simulink model "derivativemanuevermissile"  (Simulink 10.0)
settings: Solver=ode23t  StartTime=0.0  StopTime=20  RelTol=1e-3  EnableMultiTasking=on
StopFcn:
  | startplot
settings Model: Creator=Admin  LastModifiedBy=asuresh4
settings DataIOCC: LimitDataPoints=on  SignalLoggingSaveFormat=ModelDataLogs
settings OptimizationCC: ExpressionDepthLimit=2147483647
settings DebuggingCC: FcnCallInpInsideContextMsg=warning  StateNameClashWarn=warning
settings ConfigComp: CovExternalEMLEnable=off

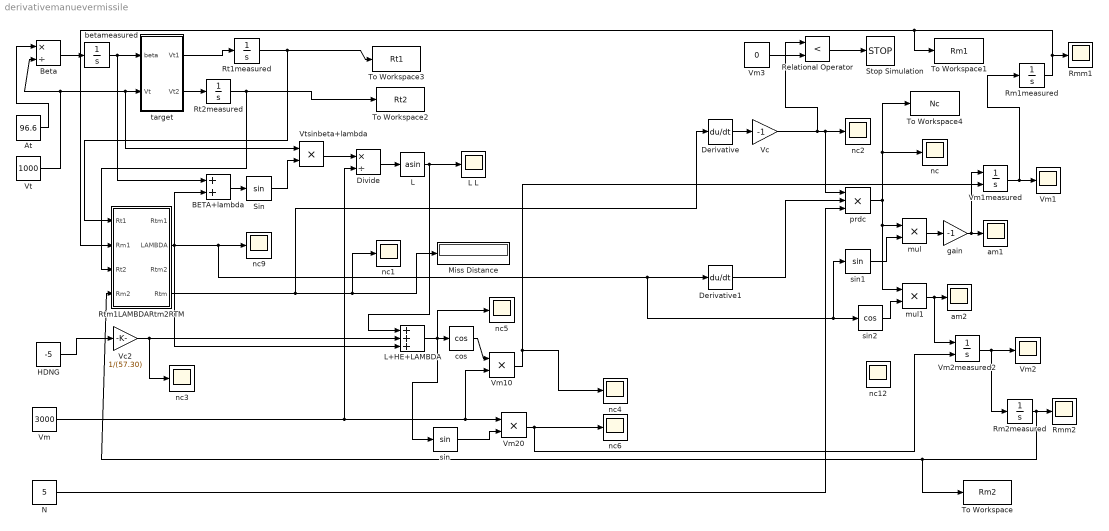
== system derivativemanuevermissile ==
  At : Constant  Value=96.6
  BETA+lambda : Sum
  Beta : Product  Inputs=*/
  Derivative : Derivative
  Derivative1 : Derivative
  Divide : Product  Inputs=*/
  HDNG : Constant  Value=-5
  L : Trigonometry  Operator=asin
  L L : Scope
  L+HE+LAMBDA : Sum  Inputs=+++
  Miss Distance : Display
  N : Constant  Value=5
  Relational Operator : RelationalOperator  Operator=<  OutDataTypeStr=boolean  SampleTime=.001  RndMeth=Nearest
  Rm1measured : Integrator
  Rm2measured : Integrator  InitialCondition=10000
  Rmm1 : Scope
  Rmm2 : Scope
  Rt1measured : Integrator  InitialCondition=40000
  Rt2measured : Integrator  InitialCondition=10000
  Rtm1LAMBDARtm2RTM : Subsystem
  Sin : Trigonometry
  Stop Simulation : Stop
  To Workspace : ToWorkspace  VariableName=Rm2  SampleTime=.01
  To Workspace1 : ToWorkspace  VariableName=Rm1  SampleTime=.01
  To Workspace2 : ToWorkspace  VariableName=Rt2  SampleTime=.01
  To Workspace3 : ToWorkspace  VariableName=Rt1  SampleTime=.01
  To Workspace4 : ToWorkspace  VariableName=Nc  SampleTime=.01
  Vc : Gain  Gain=-1
  Vc2 : Gain  Gain=1/(57.30)
  Vm : Constant  Value=3000
  Vm1 : Scope
  Vm10 : Product  RndMeth=Zero
  Vm1measured : Integrator  InitialConditionSource=external
  Vm2 : Scope
  Vm20 : Product  RndMeth=Zero
  Vm2measured2 : Integrator  InitialConditionSource=external
  Vm3 : Constant  Value=0  VectorParams1D=off
  Vt : Constant  Value=1000
  Vtsinbeta+lambda : Product  RndMeth=Zero
  am1 : Scope
  am2 : Scope
  betameasured : Integrator
  cos : Trigonometry  Operator=cos
  gain : Gain  Gain=-1
  mul : Product  Inputs=**
  mul1 : Product  Inputs=**
  nc{,1..6,9,12} (9 alike) : Scope
  prdc : Product  Inputs=***
  sin : Trigonometry
  sin1 : Trigonometry
  sin2 : Trigonometry  Operator=cos
  target : Subsystem
  wires:
  cos/1 -> Vm10/1
  sin/1 -> Vm20/2
  Vm/1 -> Divide/2, Vm20/1, Vm10/2
  BETA+lambda/1 -> Sin/1
  betameasured/1 -> target/1(beta), BETA+lambda/1
  Vt/1 -> target/2(Vt), Vtsinbeta+lambda/1, Beta/2
  Sin/1 -> Vtsinbeta+lambda/2
  Vtsinbeta+lambda/1 -> Divide/1
  Divide/1 -> L/1
  L/1 -> L+HE+LAMBDA/1, L L/1
  HDNG/1 -> Vc2/1
  L+HE+LAMBDA/1 -> sin/1, cos/1, nc5/1
  Vm10/1 -> nc4/1, Vm1measured/2
  target/1(Vt1) -> Rt1measured/1
  target/2(Vt2) -> Rt2measured/1
  Vm20/1 -> nc6/1, Vm2measured2/2
  Rtm1LAMBDARtm2RTM/2(LAMBDA) -> BETA+lambda/2, L+HE+LAMBDA/3, nc9/1, Derivative1/1, sin2/1, sin1/1
  Rtm1LAMBDARtm2RTM/4(Rtm) -> nc1/1, Miss Distance/1, Derivative/1
  Vc/1 -> Relational Operator/1, prdc/1, nc2/1
  N/1 -> prdc/3
  prdc/1 -> mul/1, mul1/1, nc/1, To Workspace4/1
  sin1/1 -> mul/2
  sin2/1 -> mul1/2
  mul/1 -> gain/1
  gain/1 -> am1/1, Vm1measured/1
  mul1/1 -> am2/1, Vm2measured2/1
  Vm1measured/1 -> Vm1/1, Rm1measured/1
  Vm2measured2/1 -> Vm2/1, Rm2measured/1
  Rm1measured/1 -> Rmm1/1, To Workspace1/1, Rtm1LAMBDARtm2RTM/2(Rm1)
  Rm2measured/1 -> Rtm1LAMBDARtm2RTM/4(Rm2), To Workspace/1, Rmm2/1
  Vc2/1 -> L+HE+LAMBDA/2, nc3/1
  Rt1measured/1 -> Rtm1LAMBDARtm2RTM/1(Rt1), To Workspace3/1
  Rt2measured/1 -> Rtm1LAMBDARtm2RTM/3(Rt2), To Workspace2/1
  At/1 -> Beta/1
  Beta/1 -> betameasured/1
  Vm3/1 -> Relational Operator/2
  Derivative/1 -> Vc/1
  Derivative1/1 -> prdc/2
  Relational Operator/1 -> Stop Simulation/1

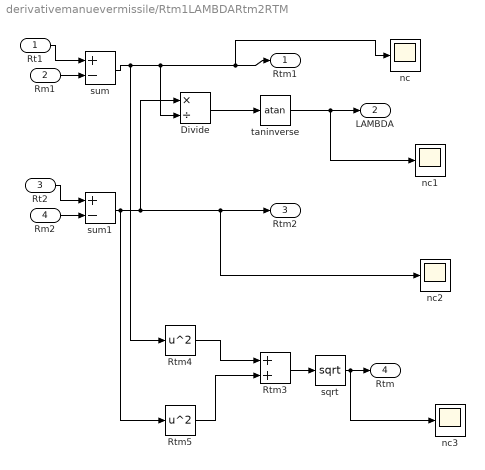
== system derivativemanuevermissile/Rtm1LAMBDARtm2RTM ==
  Rt1 : Inport
  Rm1 : Inport  Port=2
  Rt2 : Inport  Port=3
  Rm2 : Inport  Port=4
  Divide : Product  Inputs=*/
  Rtm3 : Sum
  Rtm4 : Math  Operator=square  SaturateOnIntegerOverflow=on
  Rtm5 : Math  Operator=square  SaturateOnIntegerOverflow=on
  nc{,1..3} (4 alike) : Scope
  sqrt : Math  Operator=sqrt  SaturateOnIntegerOverflow=on
  sum : Sum  Inputs=+-
  sum1 : Sum  Inputs=+-
  taninverse : Trigonometry  Operator=atan
  Rtm1 : Outport
  LAMBDA : Outport  Port=2
  Rtm2 : Outport  Port=3
  Rtm : Outport  Port=4
  wires:
  Divide/1 -> taninverse/1
  sum1/1 -> Rtm5/1, Divide/1, Rtm2/1, nc2/1
  sum/1 -> Divide/2, Rtm1/1, nc/1, Rtm4/1
  Rtm3/1 -> sqrt/1
  Rtm4/1 -> Rtm3/1
  Rtm5/1 -> Rtm3/2
  Rt1/1 -> sum/1
  Rm1/1 -> sum/2
  taninverse/1 -> LAMBDA/1, nc1/1
  Rt2/1 -> sum1/1
  Rm2/1 -> sum1/2
  sqrt/1 -> Rtm/1, nc3/1

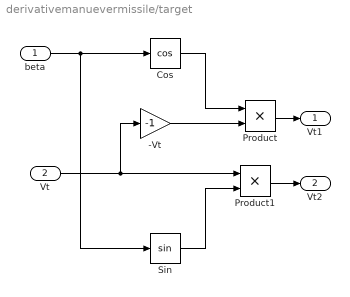
== system derivativemanuevermissile/target ==
  beta : Inport
  Vt : Inport  Port=2
  -Vt : Gain  Gain=-1
  Cos : Trigonometry  Operator=cos
  Product : Product  RndMeth=Zero
  Product1 : Product  RndMeth=Zero
  Sin : Trigonometry
  Vt1 : Outport
  Vt2 : Outport  Port=2
  wires:
  beta/1 -> Sin/1, Cos/1
  Cos/1 -> Product/1
  Sin/1 -> Product1/2
  Vt/1 -> -Vt/1, Product1/1
  -Vt/1 -> Product/2
  Product/1 -> Vt1/1
  Product1/1 -> Vt2/1
